simulink model "electric_motor"  (R2016b)
settings: Solver=FixedStepAuto  StartTime=0.0  StopTime=10.0  FixedStep=0.001  RelTol=1e-3
values from neighbouring files (symbols this model uses):
  b = 0.019029892    [motor_estimated_params.mat]    (also in motor_parameters.mat)
  beta = 0.000980862938834    [motor_estimated_params.mat]    (also in motor_parameters.mat = 0.001610902)
  J = 0.0011756012361    [motor_estimated_params.mat]    (also in motor_parameters.mat = 0.00123078313678)
  K = 0.192769478686    [motor_estimated_params.mat]    (also in motor_parameters.mat = 0.2154321312)
  R = 2.14486670574    [motor_estimated_params.mat]    (also in motor_parameters.mat = 2.4)
undefined symbols (not defined in the file): K_e, K_t
libraries: simulink x1
settings Model: Creator=piotr  LastModifiedBy=piotr

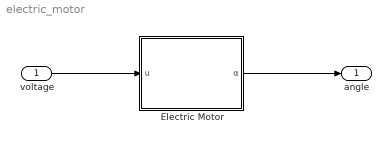
== system electric_motor ==
  voltage : Inport
  Electric Motor : Subsystem  mask{K_e=K_e, K_t=K_t, K=K, R=R, beta=beta, b=b, J=J}
      mask prompts: K_e "Electromotive force constant [V*s/rad]"; K_t "Motor torque constant [N*m/A]"; K "Motor constant"; R "Electrical resistance [Ω]"; beta "Motor viscous damping [N*m*s/rad]"; b "Motor dry damping [N*m]"; J "Motor moment of inertia [kg*m^2]"
  angle : Outport
  wires:
  voltage/1 -> Electric Motor/1(u)
  Electric Motor/1(α) -> angle/1

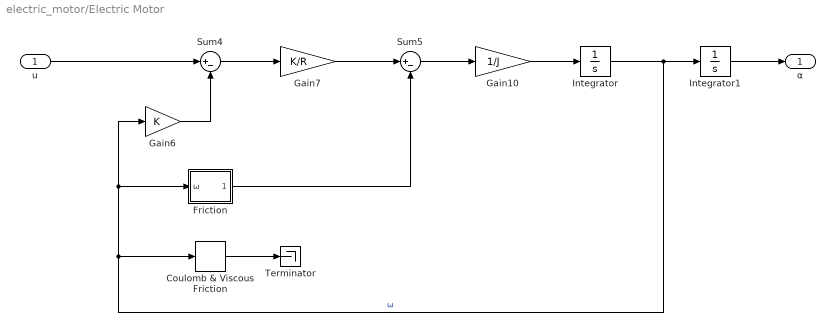
== system electric_motor/Electric Motor ==
  u : Inport
  Coulomb & Viscous Friction : simulink/Discontinuities/Coulomb & Viscous Friction  offset=beta  gain=b
  Friction : Subsystem
  Gain10 : Gain  Gain=1/J
  Gain6 : Gain  Gain=K
  Gain7 : Gain  Gain=K/R
  Integrator : Integrator
  Integrator1 : Integrator
  Sum4 : Sum  Inputs=|+-
  Sum5 : Sum  Inputs=|+-
  Terminator : Terminator
  α : Outport
  wires:
  Integrator/1 -> Integrator1/1, Coulomb & Viscous Friction/1, Gain6/1, Friction/1(ω)  "ω"
  u/1 -> Sum4/1
  Gain6/1 -> Sum4/2
  Sum4/1 -> Gain7/1
  Gain7/1 -> Sum5/1
  Sum5/1 -> Gain10/1
  Gain10/1 -> Integrator/1
  Integrator1/1 -> α/1
  Friction/1(Out1) -> Sum5/2
  Coulomb & Viscous Friction/1 -> Terminator/1

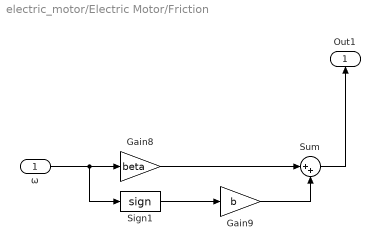
== system electric_motor/Electric Motor/Friction ==
  ω : Inport
  Gain8 : Gain  Gain=beta
  Gain9 : Gain  Gain=b
  Sign1 : Signum  ZeroCross=off
  Sum : Sum  Inputs=|++
  Out1 : Outport
  wires:
  ω/1 -> Sign1/1, Gain8/1
  Sign1/1 -> Gain9/1
  Gain8/1 -> Sum/1
  Sum/1 -> Out1/1
  Gain9/1 -> Sum/2
